simulink library "AnnLimiterBtc"  (R2022b)
settings: Solver=VariableStepAuto  StartTime=0.0  StopTime=10.0  RelTol=1e-3
undefined symbols (not defined in the file or in its folder): Column
libraries: TuneVar x8, TOP x4, AudioStats x1, FeaturePath x1, HandyTextFile x1
settings Model: Creator=kl13806  LastModifiedBy=kl13806
settings SolverCC: AlgebraicLoopSolver=TrustRegion
settings DebuggingCC: UnconnectedInputMsg=warning  UnconnectedOutputMsg=warning  UnconnectedLineMsg=warning  SFMachineParentedDataDiag=warning
settings ModelReferenceCC: EnableRefExpFcnMdlSchedulingChecks=on
settings RTWCC: DLArmComputeVersion=19.05

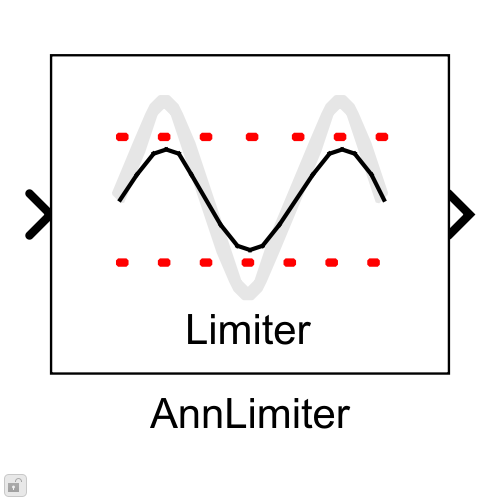
[thumbnail: Simulink's stored preview of the top-level diagram]
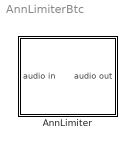
== system AnnLimiterBtc ==
  AnnLimiter : Subsystem  mask(Blocklib AnnLimiter){Config=[], FeatureName=Limiter}
      mask prompts: Config "AnnLimiterConfig"; FeatureName "Feature path name:"
      mask init:
      | blkh=gcbh;
      | Config=BTConfig.Assert(blkh,Config);
      | 
      | Config.Validate();
      | BTConfig.InitSetFeatureIfPresent(blkh,'FeatureName');
      mask Callback Config: BTConfig.CallbackHideIfPresent(gcbh,{'FeatureName'});
      mask TypeOptions FeatureName: FeaturePath/FeatureName
      mask Display:
      | [path,w,h] = IconLimiterMask();
      | 
      | % work in pixels since the icon does not scale
      | pos = get(gcbh,'position');
      | bw = pos(3) - pos(1);
      | bh = pos(4) - pos(2);
      | 
      | % Draw centered icon
      | xAdj = bw/2 - w/2;
      | yAdj = bh/2 - h/2 + 4;
      | for i=1:length(path)
      |     if (path(i).rgb(1) >= 0)
      |         patch(path(i).x+xAdj, path(i).y+yAdj, path(i).rgb);
      |     end
      |     if (path(i).stroke(1) >= 0)
      |         plot(path(i).x+xAdj, path(i).y+yAdj);
      |     end
      | end
      | 
      | % Display some text
      | text(bw/2, 4,FeatureName, ...
      |     'horizontalAlignment','center', ...
      |     'VerticalAlignment','bottom');

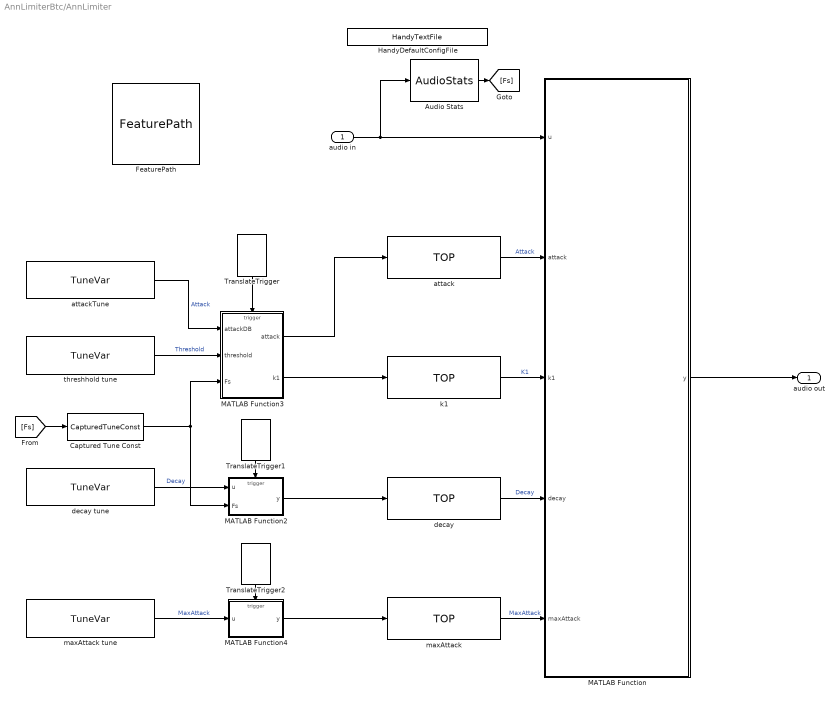
== system AnnLimiterBtc/AnnLimiter ==
  audio in : Inport
  Audio Stats : AudioStats/AudioStats  DoSampleRate=on  TypeSampleRate=double  DoCallRate=off  TypeCallRate=Inherit: auto  DoFrameSize=off  TypeFrameSize=Inherit: auto  DoChannelCount=off  TypeChannelCount=Inherit: auto  DoTaskRateFactor=off  TypeTaskRateFactor=Inherit: auto  MacroNameRoot=AUDIO  MacroNameRootEval='AUDIO'  IsMacroNameEval=off  MacroSampleRate=off  MacroCallRate=off  MacroFrameSize=off  MacroChannelCount=off  MacroTaskRateFactor=off  MacroTaskId=off  ValidateSampleRate=off  ValueSampleRate=[]  ValidateCallRate=off  ValueCallRate=[]  ValidateFrameSize=off  ValueFrameSize=[]  ValidateChannelCount=off  ValueChannelCount=[]  ValidateTaskRateFactor=off  ValueTaskRateFactor=[]
      settings: SourceProductName=Bose Talaria
  Captured Tune Const : TuneVar/CapturedTuneConst  TriggerInit=[35 527 135 563]  Role=Automatic
      settings: SourceProductName=Bose Talaria
  FeaturePath : FeaturePath/FeaturePath  FeatureName=Limiter  IsGroup=off  GroupNumber=-1  IsModule=off  TriggerInit=[95 89 210 196]
      settings: SourceProductName=Bose Talaria
  HandyDefaultConfigFile : HandyTextFile/HandyTextFile  TemplateSource=Config  FileSuffix=Init  OpenDialogOnLoad=off  UseThisBlockName=off  AddGrandParentNamePrefix=off  TheDefaultText=|  ShowInLibBrowser=on
      | % $(FILENAME) Setup model parameters for each "Init" callback (e.g. update diagram)
      | sample_rate_in_hertz = 44100;
      | frame_size = 32;
      | sysin_channel_count = 2;
      settings: SourceProductName=Bose Talaria
  MATLAB Function : MATLAB Function  TreatAsAtomicUnit=on
  MATLAB Function2 : MATLAB Function  TreatAsAtomicUnit=on
  MATLAB Function3 : MATLAB Function  TreatAsAtomicUnit=on
  MATLAB Function4 : MATLAB Function  TreatAsAtomicUnit=on
  TranslateTrigger : TuneVar/TranslateTrigger  TriggerInit=[261 290 299 345]
      settings: SourceProductName=Bose Talaria
  TranslateTrigger1 : TuneVar/TranslateTrigger  TriggerInit=[266 535 304 590]
      settings: SourceProductName=Bose Talaria
  TranslateTrigger2 : TuneVar/TranslateTrigger  TriggerInit=[266 700 304 755]
      settings: SourceProductName=Bose Talaria
  attack : TOP/TOP  TriggerInit=[460 292 610 348]  TopName=Attack  DataType=single  BankNumber=0  PreOverlay=false  PostOverlay=false  Role=Automatic
      settings: SourceProductName=Bose Talaria
  attackTune : TuneVar/TuneVar  TuneName=Attack  SpecifyMaxSize=off  VariableDim=2 (Column)  MaxSize=[1 1]  TunabilityNumber=1  MinValue=[]  MaxValue=[]  TriggerInit=[-20 325 150 375]  MaskValue=Config.DefaultAttackDb
      settings: SourceProductName=Bose Talaria
  decay : TOP/TOP  TriggerInit=[460 612 610 668]  TopName=Decay  DataType=single  BankNumber=0  PreOverlay=false  PostOverlay=false  Role=Automatic
      settings: SourceProductName=Bose Talaria
  decay tune : TuneVar/TuneVar  TuneName=Decay  SpecifyMaxSize=off  VariableDim=2 (Column)  MaxSize=[1 1]  TunabilityNumber=1  MinValue=[]  MaxValue=[]  TriggerInit=[-20 600 150 650]  MaskValue=Config.DefaultDecayDb
      settings: SourceProductName=Bose Talaria
  k1 : TOP/TOP  TriggerInit=[460 452 610 508]  TopName=K1  DataType=single  BankNumber=0  PreOverlay=false  PostOverlay=false  Role=Automatic
      settings: SourceProductName=Bose Talaria
  maxAttack : TOP/TOP  TriggerInit=[460 772 610 828]  TopName=MaxAttack  DataType=single  BankNumber=0  PreOverlay=false  PostOverlay=false  Role=Automatic
      settings: SourceProductName=Bose Talaria
  maxAttack tune : TuneVar/TuneVar  TuneName=MaxAttack  SpecifyMaxSize=off  VariableDim=2 (Column)  MaxSize=[1 1]  TunabilityNumber=1  MinValue=[]  MaxValue=[]  TriggerInit=[-20 775 150 825]  MaskValue=Config.DefaultMaxAttack
      settings: SourceProductName=Bose Talaria
  threshhold tune : TuneVar/TuneVar  TuneName=Threshold  SpecifyMaxSize=off  VariableDim=2 (Column)  MaxSize=[1 1]  TunabilityNumber=1  MinValue=[]  MaxValue=[]  TriggerInit=[-20 425 150 475]  MaskValue=Config.DefaultThreshold
      settings: SourceProductName=Bose Talaria
  audio out : Outport  VectorParamsAs1DForOutWhenUnconnected=off
  wires:
  audio in/1 -> MATLAB Function/1(u), Audio Stats/1
  MATLAB Function/1(y) -> audio out/1
  attackTune/1 -> MATLAB Function3/1(attackDB)  "Attack"
  decay tune/1 -> MATLAB Function2/1(u)  "Decay"
  TranslateTrigger1/1 -> MATLAB Function2/Trigger
  attack/1 -> MATLAB Function/2(attack)  "Attack"
  MATLAB Function2/1(y) -> decay/1
  decay/1 -> MATLAB Function/4(decay)  "Decay"
  Audio Stats/1 -> [Fs]
  [Fs] -> Captured Tune Const/1
  Captured Tune Const/1 -> MATLAB Function3/3(Fs), MATLAB Function2/2(Fs)
  threshhold tune/1 -> MATLAB Function3/2(threshold)  "Threshold"
  TranslateTrigger/1 -> MATLAB Function3/Trigger
  MATLAB Function3/2(k1) -> k1/1
  k1/1 -> MATLAB Function/3(k1)  "K1"
  maxAttack tune/1 -> MATLAB Function4/1(u)  "MaxAttack"
  TranslateTrigger2/1 -> MATLAB Function4/Trigger
  MATLAB Function4/1(y) -> maxAttack/1
  maxAttack/1 -> MATLAB Function/5(maxAttack)  "MaxAttack"
  MATLAB Function3/1(attack) -> attack/1

== matlab function AnnLimiterBtc/AnnLimiter/MATLAB Function ==
  data: u input; y output; attack input; k1 input; decay input; maxAttack input
function y = limiter(u, attack, k1, decay, maxAttack)

% Grab data from input
y = coder.nullcopy(u);
[frame_size, channel_count] = size(u);

% Initialize memory
% attack = single(2.5768580901e-002 * ones(1,channel_count));
% decay = single(1.0002610981e+000 * ones(1,channel_count));
maxGain = single(1);
% maxAttack = single(3.1622776602e-001 * ones(1,channel_count));
% k1 = single(2.8631756556e-002 * ones(1,channel_count));

persistent state;
if isempty(state)
    state = single(1 * ones(1,channel_count));
end

% Process the audio
for i = 1:channel_count
    k0 = 1 + attack(i);
    g1 = state(i);
    
    for s = 1:frame_size
        % Compute the gain for this sample. Implementation copied from BDSP
        p1 = k1(i) * g1;
        p2 = u(s, i);
        p2 = abs(p2);
        g1 = g1 * decay(i);
        p2 = p2 * p1;
        p2 = max(p2, attack(i));
        p2 = k0 - p2;
        p2 = max(p2, maxAttack(i));
        g1 = g1 * p2;
        g1 = min(g1, maxGain);
        
        % Apply the gain
        y(s, i) = u(s, i) * g1;
    end
    
    state(i) = g1;
end

== matlab function AnnLimiterBtc/AnnLimiter/MATLAB Function2 ==
  data: u input; y output; Fs input
  events: trigger input FUNCTION_CALL_EVENT
function y = fcn(u, Fs)
% convert from dB to absolute magnitude
y = single(undb20(abs(u.Value) / Fs));

== matlab function AnnLimiterBtc/AnnLimiter/MATLAB Function3 ==
  data: attackDB input; threshold input; Fs input; attack output; k1 output
  events: trigger input FUNCTION_CALL_EVENT
function [attack, k1]= fcn(attackDB, threshold, Fs)
% Compute the attack rate
attack = single(1 - undb20(-abs(attackDB.Value) / Fs));
k1 = attack ./ single(threshold.Value);

== matlab function AnnLimiterBtc/AnnLimiter/MATLAB Function4 ==
  data: u input; y output
  events: trigger input FUNCTION_CALL_EVENT
function y = fcn(u)
% Convert from dB to absolute magnitude
y = single(undb20(-abs(u.Value)));
